simulink model "simextkalman"  (R2017b)
settings: Solver=ode4  StartTime=0.0  StopTime=10.0  FixedStep=Ts  MaxStep=0.01  RelTol=1e-3  EnableMultiTasking=on
values from neighbouring files (symbols this model uses):
  b = 0.1    [funkciadynamiky.m]    (also in param.mat; simnelinkyvadlo.m; simnelinkyvadlo_mine.m)
  g = 9.81    [funkciadynamiky.m]    (also in param.mat; simnelinkyvadlo.m; simnelinkyvadlo_mine.m)
  l = 0.2    [funkciadynamiky.m]    (also in param.mat; simnelinkyvadlo.m; simnelinkyvadlo_mine.m)
  m1 = 0.4    [funkciadynamiky.m]    (also in param.mat; simnelinkyvadlo.m; simnelinkyvadlo_mine.m)
  m2 = 0.08    [funkciadynamiky.m]    (also in param.mat; simnelinkyvadlo.m; simnelinkyvadlo_mine.m)
  Ts = 0.01    [funkciadynamiky.m]    (also in kalmankyvadlo.m; simdiskkyvadlo.m; simnelinkyvadlo_mine.m; sysd.mat)
  v_var = [5e-3 5e-3]'    [simEKFkyvadlo.m]    (also in simKFkyvadlo.m)
  w_var = [0 0 0 1e-4]'    [simEKFkyvadlo.m]    (also in simKFkyvadlo.m)
  x0 = [0;0;5*pi/6;0]    [kalmankyvadlo.m]    (also in simEKFkyvadlo.m = [0;0;0;0]; simKFkyvadlo.m = [0;0;7*pi/8;0]; simnelinkyvadlo.m = [0;0;pi/6;0]; simnelinkyvadlo_mine.m = [0;0;pi/6;0])
libraries: simulink x2, sharedTrackingLibrary x1
settings Model: Creator=UAMAI-LENOVO  LastModifiedBy=gulan
settings DataIOCC: LimitDataPoints=on  SaveFormat=Array
settings OptimizationCC: LifeSpan=inf
settings DebuggingCC: SFUnexpectedBacktrackingDiag=warning  SFNoUnconditionalDefaultTransitionDiag=warning  SFExecutionAtInitializationDiag=none
settings HardwareCC: ProdBitPerPointer=32  ProdBitPerSizeT=32  ProdBitPerPtrDiffT=32  ProdLargestAtomicFloat=None  ProdIntDivRoundTo=Undefined  ProdEndianess=Unspecified  ProdWordSize=32  ProdHWDeviceType=32-bit Generic
settings ModelReferenceCC: PropagateSignalLabelsOutOfModel=off
settings CodeAppCC: StateflowObjectComments=on
settings GRTTargetCC: TargetLangStandard=C89/C90 (ANSI)  GeneratePreprocessorConditionals=Disable all
settings ConfigComp: CovMetricSettings=dw  CovHtmlReporting=on  CovSaveCumulativeToWorkspaceVar=on  CovSaveSingleToWorkspaceVar=on  CovExternalEMLEnable=off

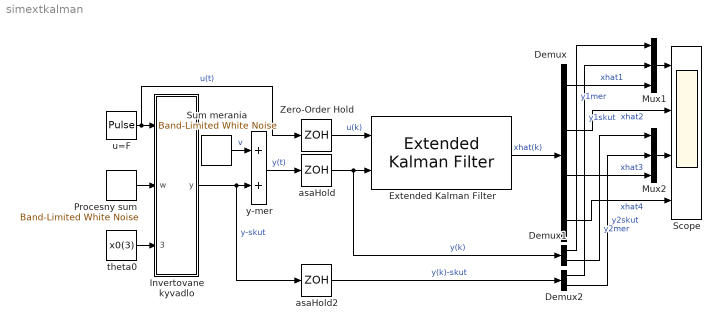
== system simextkalman ==
  " Scope" : Scope  NumInputPorts=4
  " y-mer " : Sum
  Demux : Demux
  Demux1 : Demux  Outputs=2
  Demux2 : Demux  Outputs=2
  Extended Kalman Filter : sharedTrackingLibrary/Extended Kalman Filter  StateTransitionFcn=funkciadynamiky  HasStateTransitionJacobianFcn=off  HasAdditiveProcessNoise=Additive  ProcessNoise=Q  HasTimeVaryingProcessNoise=off  HasStateTransitionFcnExtraArgument=1  InitialState=x0  InitialStateCovariance=1e0  MeasurementFcn1=funkciamerania  HasMeasurementJacobianFcn1=off  HasMeasurementEnablePort1=off  HasAdditiveMeasurementNoise1=Additive  MeasurementNoise1=R  HasTimeVaryingMeasurementNoise1=off  HasMeasurementFcnExtraArgument1=0  MeasurementFcn2=myMeasurementFcn  HasMeasurementJacobianFcn2=off  HasMeasurementEnablePort2=off  HasAdditiveMeasurementNoise2=Additive  MeasurementNoise2=1  HasTimeVaryingMeasurementNoise2=off  HasMeasurementFcnExtraArgument2=0  MeasurementFcn3=myMeasurementFcn  HasMeasurementJacobianFcn3=off  HasMeasurementEnablePort3=off  HasAdditiveMeasurementNoise3=Additive  MeasurementNoise3=1  HasTimeVaryingMeasurementNoise3=off  HasMeasurementFcnExtraArgument3=0  MeasurementFcn4=myMeasurementFcn  HasMeasurementJacobianFcn4=off  HasMeasurementEnablePort4=off  HasAdditiveMeasurementNoise4=Additive  MeasurementNoise4=1  HasTimeVaryingMeasurementNoise4=off  HasMeasurementFcnExtraArgument4=0  MeasurementFcn5=myMeasurementFcn  HasMeasurementJacobianFcn5=off  HasMeasurementEnablePort5=off  HasAdditiveMeasurementNoise5=Additive  MeasurementNoise5=1  HasTimeVaryingMeasurementNoise5=off  HasMeasurementFcnExtraArgument5=0  EnableMultirate=off  StateTransitionFcnSampleTime=1  MeasurementFcn1SampleTime=1  MeasurementFcn2SampleTime=1  MeasurementFcn3SampleTime=1  MeasurementFcn4SampleTime=1  MeasurementFcn5SampleTime=1  UseCurrentEstimator=on  OutputStateCovariance=off  DataType=double  SampleTime=Ts  NumberOfMeasurements=1
      settings: SourceProductName=Control System Toolbox  SourceProductBaseCode=CT
  Invertovane kyvadlo : Subsystem
  Mux1 : Mux  Inputs=3
  Mux2 : Mux  Inputs=3
  Procesny sum : simulink/Sources/Band-Limited White Noise  Cov=w_var*Ts*0  Ts=Ts  seed=[23341]
  Sum merania : simulink/Sources/Band-Limited White Noise  Cov=v_var*Ts  Ts=Ts  seed=[12347]
  Zero-Order Hold : ZeroOrderHold  SampleTime=Ts
  asaHold : ZeroOrderHold  SampleTime=Ts
  asaHold2 : ZeroOrderHold  SampleTime=Ts
  theta0 : Constant  Value=x0(3)  SampleTime=-1
  u=F : DiscretePulseGenerator  PulseType=Time based  Amplitude=-1  Period=10  PulseWidth=0.1  PhaseDelay=0.01
  wires:
  Zero-Order Hold/1 -> Extended Kalman Filter/1  "u(k)"
  " y-mer "/1 -> asaHold/1  "y(t)"
  Sum merania/1 -> " y-mer "/1  "v"
  Procesny sum/1 -> Invertovane kyvadlo/2(w)
  u=F/1 -> Zero-Order Hold/1, Invertovane kyvadlo/1(u)  "u(t)"
  Invertovane kyvadlo/1(y) -> " y-mer "/2, asaHold2/1  "y-skut"
  theta0/1 -> Invertovane kyvadlo/3(theta0)
  asaHold/1 -> Demux1/1, Extended Kalman Filter/2  "y(k)"
  Demux2/2 -> Mux2/2  "y2skut"
  Demux1/2 -> Mux2/1  "y2mer"
  Demux2/1 -> Mux1/2  "y1skut"
  Demux1/1 -> Mux1/1  "y1mer"
  Demux/4 -> " Scope"/4  "xhat4"
  Demux/2 -> " Scope"/2  "xhat2"
  Mux1/1 -> " Scope"/1
  Demux/3 -> Mux2/3  "xhat3"
  Mux2/1 -> " Scope"/3
  Extended Kalman Filter/1 -> Demux/1  "xhat(k)"
  Demux/1 -> Mux1/3  "xhat1"
  asaHold2/1 -> Demux2/1  "y(k)-skut"

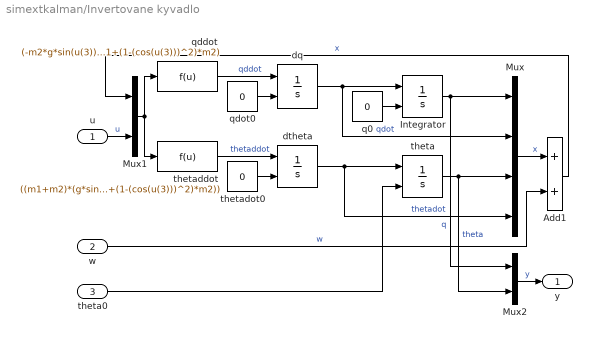
== system simextkalman/Invertovane kyvadlo ==
  u : Inport
  w : Inport  Port=2
  theta0 : Inport  Port=3
  Add1 : Sum
  Integrator : Integrator  InitialConditionSource=external
  Mux : Mux
  Mux1 : Mux  Inputs=2
  Mux2 : Mux  Inputs=2
  dq : Integrator  InitialConditionSource=external
  dtheta : Integrator  InitialConditionSource=external
  q0 : Constant  Value=0
  qddot : Fcn  Expr=(-m2*g*sin(u(3))*cos(u(3))+m2*l*((u(4))^2)*sin(u(3))+b*m2*u(4)*cos(u(3))+u(5))/(m1+(1-(cos(u(3)))^2)*m2)
  qdot0 : Constant  Value=0
  theta : Integrator  InitialConditionSource=external
  thetaddot : Fcn  Expr=((m1+m2)*(g*sin(u(3))-b*u(4))-(m2*l*((u(4))^2)*sin(u(3))+u(5))*cos(u(3)))/(l*(m1+(1-(cos(u(3)))^2)*m2))
  thetadot0 : Constant  Value=0
  y : Outport
  wires:
  dq/1 -> Mux/2, Integrator/1  "qdot"
  dtheta/1 -> Mux/4, theta/1  "thetadot"
  Integrator/1 -> Mux/1, Mux2/1  "q"
  theta/1 -> Mux/3, Mux2/2  "theta"
  qddot/1 -> dq/1  "qddot"
  thetaddot/1 -> dtheta/1  "thetaddot"
  qdot0/1 -> dq/2
  q0/1 -> Integrator/2
  thetadot0/1 -> dtheta/2
  Mux/1 -> Add1/1  "x"
  Mux1/1 -> thetaddot/1, qddot/1
  theta0/1 -> theta/2
  Mux2/1 -> y/1  "y"
  u/1 -> Mux1/2  "u"
  w/1 -> Add1/2  "w"
  Add1/1 -> Mux1/1  "x"
